simulink model "sml_driveline"  (R2016a)
settings: Solver=VariableStepAuto  StartTime=0.0  StopTime=10.0  RelTol=1e-3
libraries: simulink x1
settings Model: Creator=Duy Nam  LastModifiedBy=Duy Nam

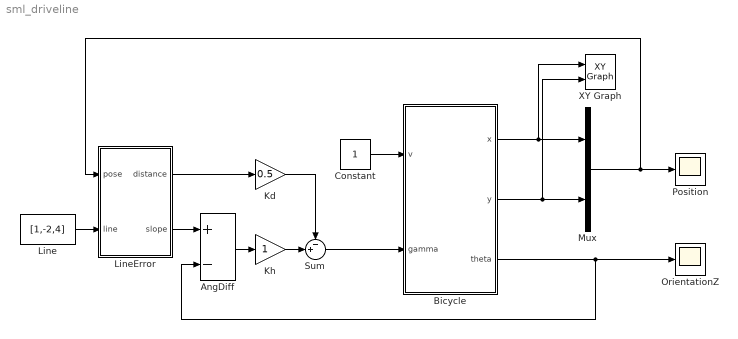
== system sml_driveline ==
  AngDiff : Sum  Inputs=+-
  Bicycle : Subsystem
  Constant : Constant
  Kd : Gain  Gain=0.5
  Kh : Gain
  Line : Constant  Value=[1,-2,4]
  LineError : MATLAB Function  TreatAsAtomicUnit=on
  Mux : Mux  Inputs=2
  OrientationZ : Scope
  Position : Scope
  Sum : Sum  Inputs=-+|
  XY Graph : simulink/Sinks/XY Graph  xmin=0  xmax=10  ymin=0  ymax=10  st=-1
  wires:
  Bicycle/2(y) -> XY Graph/2, Mux/2
  Bicycle/1(x) -> XY Graph/1, Mux/1
  Bicycle/3(theta) -> AngDiff/2, OrientationZ/1
  Mux/1 -> LineError/1(pose), Position/1
  Constant/1 -> Bicycle/1(v)
  Line/1 -> LineError/2(line)
  LineError/1(distance) -> Kd/1
  LineError/2(slope) -> AngDiff/1
  AngDiff/1 -> Kh/1
  Kh/1 -> Sum/2
  Kd/1 -> Sum/1
  Sum/1 -> Bicycle/2(gamma)

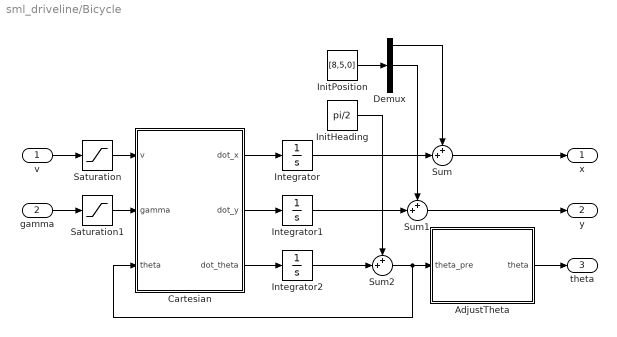
== system sml_driveline/Bicycle ==
  v : Inport
  gamma : Inport  Port=2
  AdjustTheta : MATLAB Function  TreatAsAtomicUnit=on
  Cartesian : MATLAB Function  TreatAsAtomicUnit=on
  Demux : Demux  Outputs=3
  InitHeading : Constant  Value=pi/2
  InitPosition : Constant  Value=[8,5,0]
  Integrator : Integrator
  Integrator1 : Integrator
  Integrator2 : Integrator
  Saturation : Saturate  UpperLimit=1  LowerLimit=-1
  Saturation1 : Saturate  UpperLimit=2  LowerLimit=-2
  Sum : Sum  Inputs=++|
  Sum1 : Sum  Inputs=++|
  Sum2 : Sum  Inputs=++|
  x : Outport
  y : Outport  Port=2
  theta : Outport  Port=3
  wires:
  Cartesian/1(dot_x) -> Integrator/1
  Integrator/1 -> Sum/2
  Cartesian/2(dot_y) -> Integrator1/1
  v/1 -> Saturation/1
  Integrator1/1 -> Sum1/2
  Cartesian/3(dot_theta) -> Integrator2/1
  gamma/1 -> Saturation1/1
  AdjustTheta/1(theta) -> theta/1
  Sum2/1 -> Cartesian/3(theta), AdjustTheta/1(theta_pre)
  Saturation/1 -> Cartesian/1(v)
  Saturation1/1 -> Cartesian/2(gamma)
  InitPosition/1 -> Demux/1
  Sum/1 -> x/1
  Demux/1 -> Sum/1
  Sum1/1 -> y/1
  Demux/2 -> Sum1/1
  Integrator2/1 -> Sum2/2
  InitHeading/1 -> Sum2/1

== matlab function sml_driveline/Bicycle/AdjustTheta ==
  data: theta_pre input; theta output
function theta = AdjustTheta(theta_pre)
% ADJUSTTHETA Adjust the heading angle always between [-pi/2;pi/2]
%% INPUTS
% theta_pre = The heading angle before adjust
%% OUTPUTS
% theta = The heading angle after adjust
%% Adjust Theta
theta = theta_pre - 2*pi*floor((theta_pre + pi)/(2*pi));
end

== matlab function sml_driveline/Bicycle/Cartesian ==
  data: dot_x output; dot_y output; v input; gamma input; theta input; dot_theta output
function [dot_x, dot_y, dot_theta] = Cartesian(v, gamma, theta)
% CARTESIAN Compute the velocity of robot in world frame
%% INPUTS
% v     = The velocity of the back wheel
% gamma = The steering wheel angle
% theta = The heading angle
%% OUTPUTS
% dot_x     = The velocity of robot in world frame x-axis
% dot_y     = The velocity of robot in world frame y-axis
% dot_theta = The rate of change of heading
%% Parameters
L = params_bicycle();
%% Cartesian
dot_x = v*cos(theta);
dot_y = v*sin(theta);
dot_theta = v/L*tan(gamma);
end

== matlab function sml_driveline/LineError ==
  data: pose input; distance output; line input; slope output
function [distance, slope] = LineError(pose, line)
% LINEERROR Compute distance and heading angle from Robot to Line
%% INPUTS
% pose = The current position (x, y) of Robot
% line = The target line which robot have to moving to (ax+by+c=0)
%% OUTPUTS
% distance  = The distance from Robot to the line
% slope     = The heading angle
%% Define the parameters
a = line(1); b = line(2); c = line(3);
x = pose(1); y = pose(2);
%% Compute
distance = (a*x + b*y + c)/sqrt(a^2 + b^2);
slope = atan2(-a,b);
end
